simulink model "car_control_3d"  (R2023a)
settings: Solver=VariableStepAuto  StartTime=0.0  StopTime=inf  RelTol=1e-3
values from neighbouring files (symbols this model uses):
  m = 2.5    [car_control.mat]
  r = 0.15    [car_control.mat]
libraries: vrlib x1
settings Model: Creator=The MathWorks, Inc.  LastModifiedBy=15113
settings SolverCC: AlgebraicLoopSolver=TrustRegion
settings DataIOCC: ReturnWorkspaceOutputs=off
settings OptimizationCC: ReuseModelBlockBuffer=off
settings DebuggingCC: BusObjectLabelMismatch=none  RootOutportRequireBusObject=none  PregeneratedLibrarySubsystemCodeDiagnostic=none  ArithmeticOperatorsInVariantConditions=warning
settings ModelReferenceCC: EnableRefExpFcnMdlSchedulingChecks=on
settings SFSimCC: SimUseLocalCustomCode=off
settings RTWCC: RTWUseLocalCustomCode=off

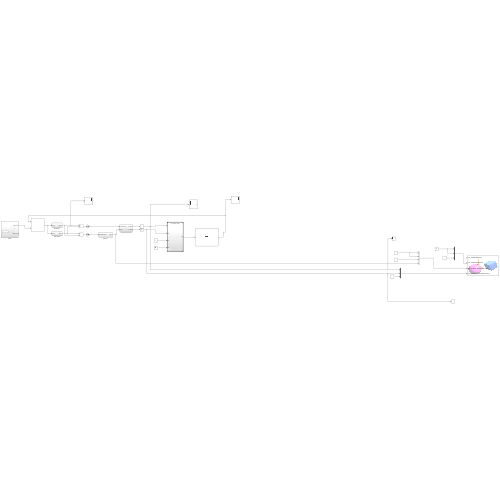
[thumbnail: Simulink's stored preview of the top-level diagram]
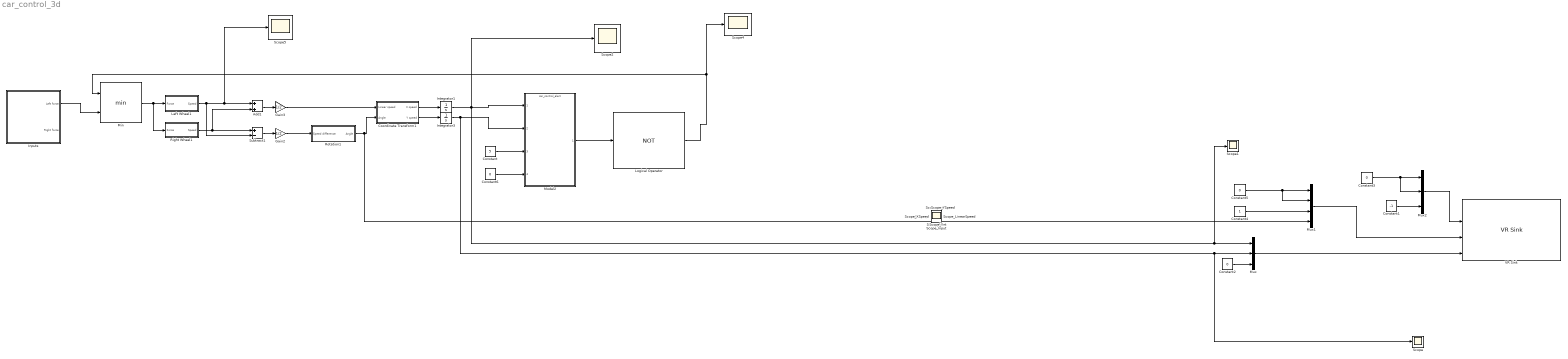
== system car_control_3d ==
  Add1 : Sum
  Constant : Constant  Value=5
  Constant1 : Constant  Value=-1
  Constant{2..3,5..6} (4 alike) : Constant  Value=0
  Constant4 : Constant
  Coordinate Transform1 : Subsystem
  Gain2 : Gain  Gain=1/2
  Gain3 : Gain  Gain=1/2
  Inputs : Subsystem
  Integrator1 : Integrator
  Integrator3 : Integrator
  Left Wheel1 : Subsystem
  Logical Operator : Logic  Operator=NOT  AllPortsSameDT=off  OutDataTypeStr=boolean
  Min : MinMax  Inputs=2
  Model2 : ModelReference  ModelNameDialog=car_control_alert.slx  SimulationMode=Normal  ModelReferenceVersion=1.5
  Mux : Mux  Inputs=3
  Mux1 : Mux
  Mux2 : Mux  Inputs=3
  Right Wheel1 : Subsystem
  Rotation1 : Subsystem
  Scope{,1..2,4..5} (5 alike) : Scope
  Subtract1 : Sum  Inputs=+-
  VR Sink : vrlib/VR Sink  InstantiateOnLoad=on  SampleTime=0.1  ViewEnable=on  RemoteChange=off  RemoteView=off  FieldsWritten=Cube_TRANSFORM.rotation.4.1.1.double#Cube_TRANSFORM.translation.3.1.1.double#Sedan_SkelMesh_TRANSFORM.rotation.4.1.1.double#Sedan_SkelMesh_TRANSFORM.translation.3.1.1.double  WorldFileName=carWithBackground.x3d  AutoView=off  VideoDimensions=[]  AllowVariableSize=off
  Scope_Alert : Scope
  Scope_Angle : Scope
  Scope_Input : Scope
  Scope_LinearSpeed : Scope
  Scope_X : Scope
  Scope_XSpeed : Scope
  Scope_Y : Scope
  Scope_YSpeed : Scope
  wires:
  Integrator1/1 -> Scope1/1, Mux/1, Scope2/1, Model2/1
  Integrator3/1 -> Scope/1, Mux/2, Model2/2
  Constant3/1 -> Mux2/2, Mux2/1
  Constant5/1 -> Mux1/2, Mux1/1
  Constant2/1 -> Mux/3
  Constant4/1 -> Mux1/3
  Mux2/1 -> VR Sink/2
  Mux1/1 -> VR Sink/3
  Mux/1 -> VR Sink/4
  Constant1/1 -> Mux2/3
  Constant/1 -> Model2/3
  Gain2/1 -> Rotation1/1(Speed difference)
  Subtract1/1 -> Gain2/1
  Add1/1 -> Gain3/1
  Gain3/1 -> Coordinate Transform1/1(Linear speed)
  Coordinate Transform1/2(Y speed) -> Integrator3/1
  Coordinate Transform1/1(X speed) -> Integrator1/1
  Left Wheel1/1(Speed) -> Subtract1/2, Scope5/1, Add1/1
  Min/1 -> Right Wheel1/1(Force), Left Wheel1/1(Force)
  Rotation1/1(Angle) -> Mux1/4, Coordinate Transform1/2(Angle)
  Right Wheel1/1(Speed) -> Add1/2, Subtract1/1
  Constant6/1 -> Model2/4
  Inputs/1(Left force) -> Min/2
  Model2/1 -> Logical Operator/1
  Logical Operator/1 -> Min/1, Scope4/1

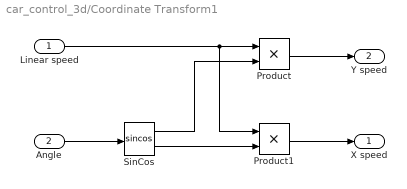
== system car_control_3d/Coordinate Transform1 ==
  Linear speed : Inport
  Angle : Inport  Port=2
  Product : Product
  Product1 : Product
  SinCos : Trigonometry  Operator=sincos
  X speed : Outport  VectorParamsAs1DForOutWhenUnconnected=off
  Y speed : Outport  Port=2  VectorParamsAs1DForOutWhenUnconnected=off
  wires:
  Angle/1 -> SinCos/1
  SinCos/2 -> Product1/2
  SinCos/1 -> Product/2
  Linear speed/1 -> Product/1, Product1/1
  Product/1 -> Y speed/1
  Product1/1 -> X speed/1

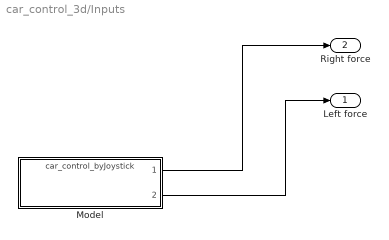
== system car_control_3d/Inputs ==
  Model : ModelReference  ModelNameDialog=car_control_byJoystick.slx  SimulationMode=Normal  ModelReferenceVersion=1.4
  Left force : Outport  VectorParamsAs1DForOutWhenUnconnected=off
  Right force : Outport  Port=2  VectorParamsAs1DForOutWhenUnconnected=off
  wires:
  Model/1 -> Right force/1
  Model/2 -> Left force/1

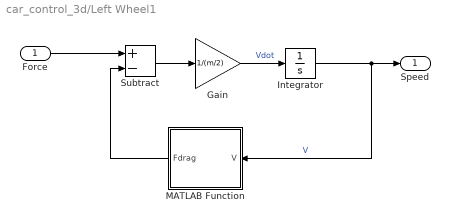
== system car_control_3d/Left Wheel1 ==
  Force : Inport
  Gain : Gain  Gain=1/(m/2)
  Integrator : Integrator
  MATLAB Function : MATLAB Function  TreatAsAtomicUnit=on
  Subtract : Sum  Inputs=+-
  Speed : Outport  VectorParamsAs1DForOutWhenUnconnected=off
  wires:
  MATLAB Function/1(Fdrag) -> Subtract/2
  Subtract/1 -> Gain/1
  Gain/1 -> Integrator/1  "Vdot"
  Integrator/1 -> MATLAB Function/1(V), Speed/1  "V"
  Force/1 -> Subtract/1

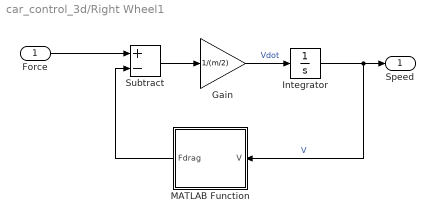
== system car_control_3d/Right Wheel1 ==
  Force : Inport
  Gain : Gain  Gain=1/(m/2)
  Integrator : Integrator
  MATLAB Function : MATLAB Function  TreatAsAtomicUnit=on
  Subtract : Sum  Inputs=+-
  Speed : Outport  VectorParamsAs1DForOutWhenUnconnected=off
  wires:
  Integrator/1 -> MATLAB Function/1(V), Speed/1  "V"
  Subtract/1 -> Gain/1
  MATLAB Function/1(Fdrag) -> Subtract/2
  Gain/1 -> Integrator/1  "Vdot"
  Force/1 -> Subtract/1

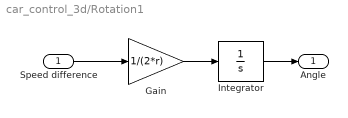
== system car_control_3d/Rotation1 ==
  Speed difference : Inport
  Gain : Gain  Gain=1/(2*r)
  Integrator : Integrator
  Angle : Outport  VectorParamsAs1DForOutWhenUnconnected=off
  wires:
  Integrator/1 -> Angle/1
  Speed difference/1 -> Gain/1
  Gain/1 -> Integrator/1

== matlab function car_control_3d/Right Wheel1/MATLAB Function ==
  data: V input; Fdrag output; k_drag parameter
function Fdrag = get_fdrag(V,k_drag)

Fdrag = k_drag*V*abs(V);

== matlab function car_control_3d/Left Wheel1/MATLAB Function ==
  data: V input; Fdrag output; k_drag parameter
function Fdrag = get_fdrag(V,k_drag)

Fdrag = k_drag*V*abs(V);
